simulink model "schema_fonctionnel_1"  (R2021b)
settings: Solver=VariableStepAuto  StartTime=0.0  StopTime=0.5  RelTol=1e-3
values from neighbouring files (symbols this model uses):
  Jt = 2*J0 + Ja2    (= 5.6e-06)    [data.m]    (also in data2.m)
  kc = 0.022    [data.m]    (also in data2.m)
  kcm = 1    [data.m]    (also in data2.m)
  kp = 1    [data.m]    (also in data2.m = 8)
  ku = 0.022    [data.m]    (also in data2.m)
  La = 10e-6    (= 1e-05)    [data.m]    (also in data2.m)
  mr = 5e-3    (= 0.005)    [data.m]    (also in data2.m)
  Ra = 5.4    [data.m]    (also in data2.m)
  s1 = -50    [data2.m]
undefined symbols (not defined in the file or in its folder): s
settings Model: Creator=gaeta  LastModifiedBy=gaeta

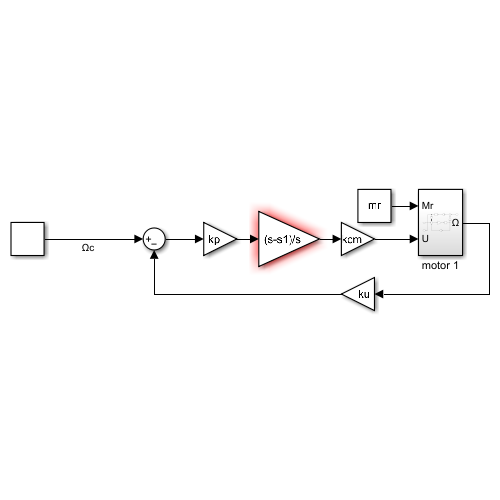
[thumbnail: Simulink's stored preview of the top-level diagram]
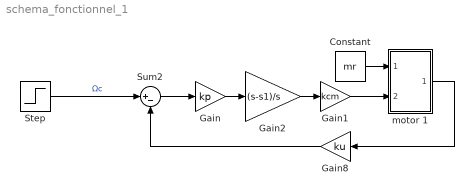
== system schema_fonctionnel_1 ==
  Constant : Constant  Value=mr
  Gain : Gain  Gain=kp
  Gain1 : Gain  Gain=kcm
  Gain2 : Gain  Gain=(s-s1)/s
  Gain8 : Gain  Gain=ku
  Step : Step  Time=0  After=2600*2*pi/60*ku  SampleTime=0
  Sum2 : Sum  Inputs=|+-
  motor 1 : Subsystem
  wires:
  Sum2/1 -> Gain/1
  Constant/1 -> motor 1/1(In1)
  motor 1/1(Out2) -> Gain8/1
  Step/1 -> Sum2/1  "Ωc"
  Gain8/1 -> Sum2/2
  Gain1/1 -> motor 1/2(In2)
  Gain/1 -> Gain2/1
  Gain2/1 -> Gain1/1

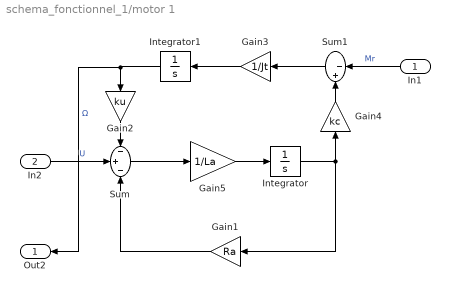
== system schema_fonctionnel_1/motor 1 ==
  In1 : Inport
  In2 : Inport  Port=2
  Gain1 : Gain  Gain=Ra
  Gain2 : Gain  Gain=ku
  Gain3 : Gain  Gain=1/Jt
  Gain4 : Gain  Gain=kc
  Gain5 : Gain  Gain=1/La
  Integrator : Integrator  LimitOutput=on  UpperSaturationLimit=2  LowerSaturationLimit=-2
  Integrator1 : Integrator
  Sum : Sum  Inputs=-+-
  Sum1 : Sum  Inputs=|-+
  Out2 : Outport
  wires:
  Gain5/1 -> Integrator/1
  Gain1/1 -> Sum/3
  Sum/1 -> Gain5/1
  Sum1/1 -> Gain3/1
  Integrator/1 -> Gain4/1, Gain1/1
  In2/1 -> Sum/2  "U"
  Integrator1/1 -> Out2/1, Gain2/1  "Ω"
  Gain2/1 -> Sum/1
  Gain3/1 -> Integrator1/1
  In1/1 -> Sum1/1  "Mr"
  Gain4/1 -> Sum1/2
